simulink model "Relay"  (R2022a)
settings: Solver=FixedStepAuto  StartTime=0.0  StopTime=30  FixedStep=0.1  RelTol=1e-3
values from neighbouring files (symbols this model uses):
  td = ((PM - 37)/(360))* Tc    (= 0.0116666666667)    [pid_relay.m]
settings Model: Creator=josed  LastModifiedBy=josed

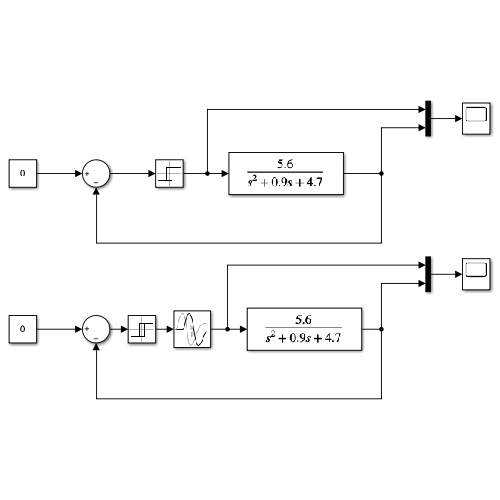
[thumbnail: Simulink's stored preview of the top-level diagram]
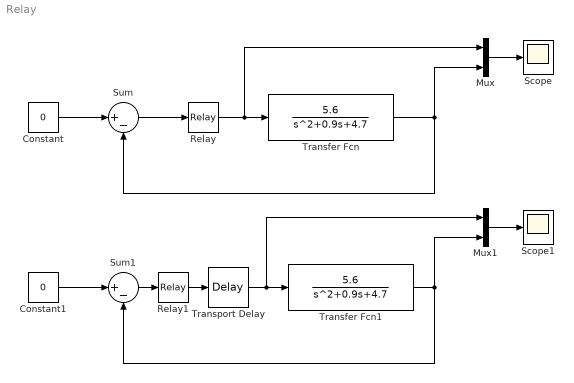
== system Relay ==
  Constant : Constant  Value=0
  Constant1 : Constant  Value=0
  Mux : Mux  Inputs=2
  Mux1 : Mux  Inputs=2
  Relay : Relay  OffOutputValue=-1
  Relay1 : Relay  OffOutputValue=-1
  Scope : Scope
  Scope1 : Scope
  Sum : Sum  Inputs=|+-
  Sum1 : Sum  Inputs=|+-
  Transfer Fcn : TransferFcn  Numerator=[5.6]  Denominator=[1 0.9 4.7]
  Transfer Fcn1 : TransferFcn  Numerator=[5.6]  Denominator=[1 0.9 4.7]
  Transport Delay : TransportDelay  DelayTime=td
  wires:
  Sum/1 -> Relay/1
  Constant/1 -> Sum/1
  Relay/1 -> Mux/1, Transfer Fcn/1
  Transfer Fcn/1 -> Mux/2, Sum/2
  Mux/1 -> Scope/1
  Mux1/1 -> Scope1/1
  Transfer Fcn1/1 -> Mux1/2, Sum1/2
  Constant1/1 -> Sum1/1
  Relay1/1 -> Transport Delay/1
  Sum1/1 -> Relay1/1
  Transport Delay/1 -> Mux1/1, Transfer Fcn1/1
